simulink model "Q1e"  (R2021b)
settings: Solver=VariableStepAuto  StartTime=0.0  StopTime=16  RelTol=1e-3
undefined symbols (not defined in the file or in its folder): sigbuilder_block
libraries: dspsrcs4 x2, simulink_extras x1
settings Model: Creator=adamj  LastModifiedBy=adamj

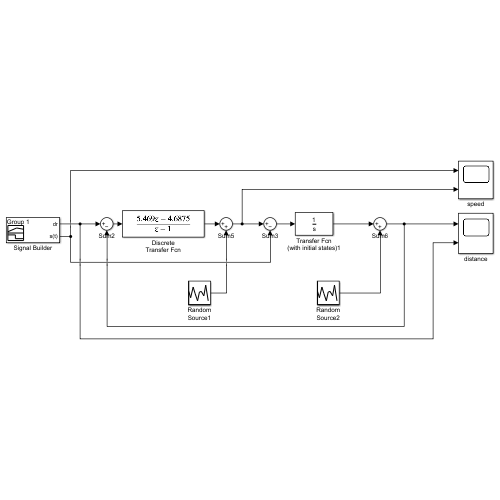
[thumbnail: Simulink's stored preview of the top-level diagram]
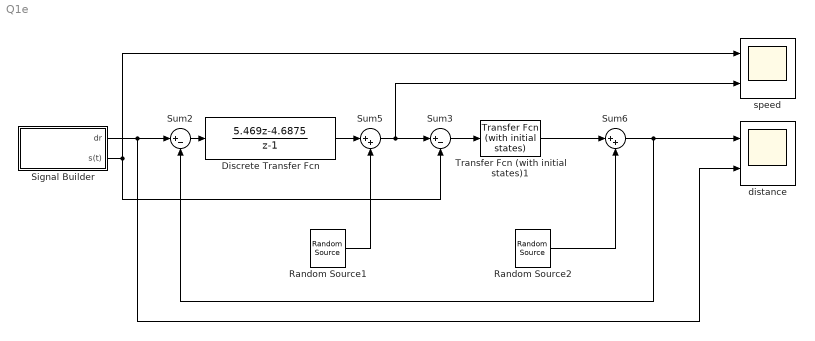
== system Q1e ==
  Discrete Transfer Fcn : DiscreteTransferFcn  Numerator=[5.469 -4.6875]  Denominator=[1 -1]  SampleTime=0.2
  Random Source1 : dspsrcs4/Random Source  SrcType=Gaussian  NormMethod=Ziggurat  CltLength=12  MinVal=0  MaxVal=1  MeanVal=0  VarVal=0.0001  RepMode=Repeatable  rawSeed=1  IsInherit=off  SampMode=Discrete  SampTime=0.2  SampFrame=1  DataType=Double  OutComplex=Real  OutputFrames=off
  Random Source2 : dspsrcs4/Random Source  SrcType=Gaussian  NormMethod=Ziggurat  CltLength=12  MinVal=0  MaxVal=1  MeanVal=0  VarVal=0.0001  RepMode=Repeatable  rawSeed=1  IsInherit=off  SampMode=Discrete  SampTime=0.2  SampFrame=1  DataType=Double  OutComplex=Real  OutputFrames=off
  Signal Builder : Subsystem  Tag=STV Subsys  LoadFcn=sigbuilder_block('load');  StartFcn=sigbuilder_block('start');  StopFcn=sigbuilder_block('stop');  ClipboardFcn=sigbuilder_block('clipboard');  mask(Sigbuilder block){tuvar=[0:10]}
      mask help: Simulink:masks:SigbuilderBlock_MD
      mask init:
      | if ~strcmp(get_param(bdroot(gcbh),'SimulationStatus'),'stopped') tuvar = sigbuilder_block('maskInit'); end
      settings: CopyFcn=sigbuilder_block('copy');  DeleteFcn=sigbuilder_block('delete');  ModelCloseFcn=sigbuilder_block('modelClose');  PreSaveFcn=sigbuilder_block('preSave');  PauseFcn=sigbuilder_block('pause');  ContinueFcn=sigbuilder_block('continue');  NameChangeFcn=sigbuilder_block('namechange');  OpenFcn=sigbuilder_block('open',[591 115.8 555.6 244.2 ]);  CloseFcn=sigbuilder_block('close');
      mask Display: plot(0, 0, 100, 100,[2, 2, 32, 32, 2], [68, 8, 8, 68, 68],[32, 2], [38, 38], [32, 19, 2],[53, 60, 44], [32, 17, 17, 2],[16, 16, 31, 31]);txt = getActiveGroup(gcbh);text(2, 100, txt,'verticalAlignment', 'top');
  Sum2 : Sum  Inputs=|+-
  Sum3 : Sum  Inputs=|+-
  Sum5 : Sum  Inputs=|++
  Sum6 : Sum  Inputs=|++
  Transfer Fcn (with initial states)1 : simulink_extras/Additional Linear/Transfer Fcn (with initial states)  N=[0 1]  D="[1  0]"  X0=1
  distance : Scope  NumInputPorts=2
  speed : Scope  NumInputPorts=2
  wires:
  Signal Builder/2(s(t)) -> Sum3/2, speed/1
  Signal Builder/1(dr) -> distance/2, Sum2/1
  Sum2/1 -> Discrete Transfer Fcn/1
  Sum3/1 -> Transfer Fcn (with initial states)1/1
  Transfer Fcn (with initial states)1/1 -> Sum6/1
  Random Source1/1 -> Sum5/2
  Sum5/1 -> speed/2, Sum3/1
  Discrete Transfer Fcn/1 -> Sum5/1
  Random Source2/1 -> Sum6/2
  Sum6/1 -> distance/1, Sum2/2

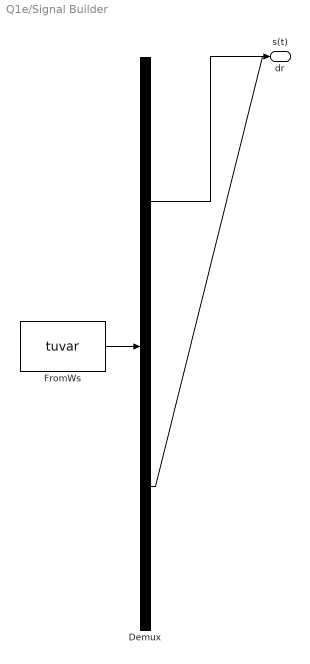
== system Q1e/Signal Builder ==
  Demux : Demux  Tag=STV Demux  Outputs=2
      settings: DisplayOption=none
  FromWs : FromWorkspace  Tag=STV FromWs  VariableName=tuvar
      SigBuilderData=|
      | common.afterFinalStr = 'Extrapolate'
      | common.sampleTime = 0
      | dataSet.timeRange = [0 50]
      | dataSet.name = 'Group 1'
      | sbobj.Groups.Name = 'Group 1'
      | sbobj.Groups.Signals(1).Name = 'dr'
      | sbobj.Groups.Signals(1).XData = [0 50]
      | sbobj.Groups.Signals(1).YData = [1 1]
      | sbobj.Groups.Signals(2).Name = 's(t)'
      | sbobj.Groups.Signals(2).XData = [0 4 8 12 30 50]
      | sbobj.Groups.Signals(2).YData = [0 0.4 0.4 0.2 0.2 0.2]
      | sbobj.Groups.TimeRange = [0 50]
  dr : Outport  Tag=STV Outport
  s(t) : Outport  Tag=STV Outport  Port=2
  wires:
  FromWs/1 -> Demux/1
  Demux/1 -> dr/1
  Demux/2 -> s(t)/1
